simulink model "TRAMI_DCT_AT"  (R2018b)
settings: Solver=FixedStepDiscrete  StartTime=0.0  StopTime=88  FixedStep=10e-3  RelTol=1e-3  EnableMultiTasking=on
undefined symbols (not defined in the file): CONST_AP_GEAR_SUB_NEWTRAL, CONST_AP_IDLE_SPEED_CONT, CONST_AP_LOAD_SFT, CONST_AP_LOAD_SFT_HYS, CONST_CAR_WEIGHT, CONST_CL_NUM, CONST_F_DOWN_SYNCHRO, CONST_F_SYNCHRO, CONST_F_UP_SYNCHRO, CONST_FGR, CONST_I_FlYWHEEL, CONST_INATIA_CLANK, CONST_R_SHIFT_END_CD, CONST_R_SHIFT_END_EG, CONST_R_SHIFT_END_TD, CONST_R_SHIFT_END_UP, CONST_R_SYNCHRO_ENGAGE, CONST_R_TIRE, CONST_RATIO_TQ_REDUCTION, CONST_SKIP_SHIFT_MAX, CONST_SYN_NUM, CONST_T_SFT_END_EN, CONST_T_SFT_END_JUDGE, CONST_T_SFT_END_MAX, CONST_T_SFT_END_MIN, CONST_T_SHIFT_WAIT, CONST_T_TQ_PHASE_CD, CONST_T_TQ_PHASE_ND, CONST_T_TQ_PHASE_NR, CONST_T_TQ_PHASE_TD, CONST_T_TQ_PHASE_UP, CONST_TQ_CREEP_CONT, CONST_TQ_ENGAGE_CL_MARGIN, CONST_TQ_ENGAGE_CL_MIN, CONST_TQ_INATIA_TD_SHIFT, CONST_TQ_LOAD_SFT, CONST_TQ_LOAD_SFT_HYS, CONST_TQ_ND_ENGAGE, CONST_TQ_NR_ENGAGE, CONST_TQ_TQPHASE_MIN, CONST_V_IDLE_SPEED_CONT, Eng, FALSE, GrNP, GrRev, LoopTime, MAT_CL_ENGAGE, MAT_CL_SHARE_RATE, MAT_I_ACTUATOR, MAT_SYNCHRO_COM, MAT_T_GEAR_SUB_NEWTRAL, MAT_TRANS_MGR, MaxCL, Nm, PI, Shift_CD, Shift_ND, Shift_NR, Shift_TD, Shift_Up ... (+168)
libraries: simulink x26
(part 3 of 6)

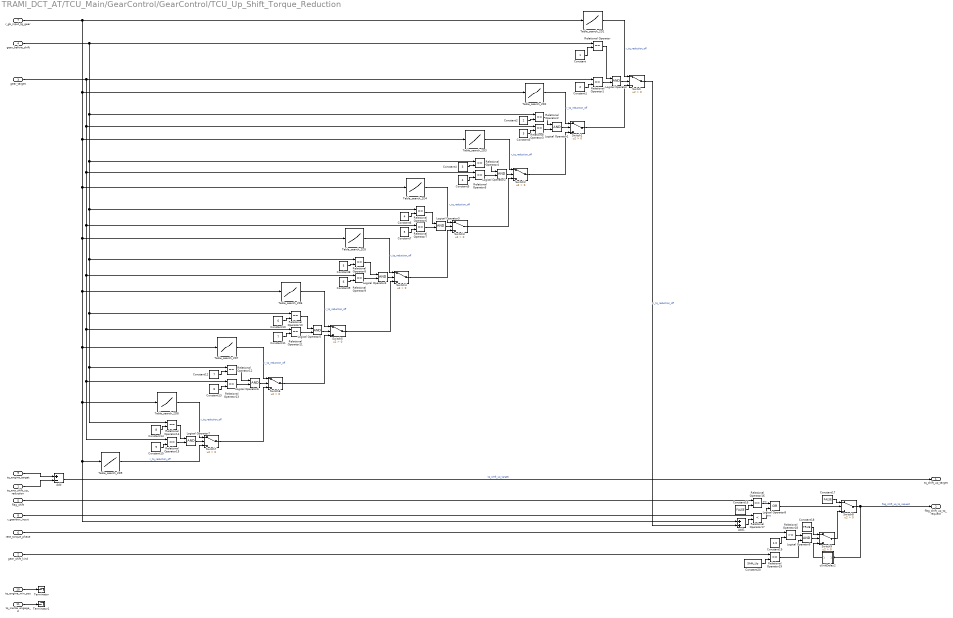
== system TRAMI_DCT_AT/TCU_Main/GearControl/GearControl/TCU_Up_Shift_Torque_Reduction ==
  tq_eng_shift_up_reduction : Inport  OutDataTypeStr=single
      settings: AttributesFormatString=アップシフト時のエンジントルクリダクション量[Nm]
  gear_shift_kind : Inport  Port=2  OutDataTypeStr=int16
      settings: AttributesFormatString=|
      | ギヤ変速種別
      | 5 : N->R
      | 4 : N->D
      | 3 : Torque demand shift
      | 2 : Coast down shift
      | 1 : Schedule up shift
      | [-]
  gear_target : Inport  Port=3  OutDataTypeStr=int16
      settings: AttributesFormatString=目標ギヤ段[-]
  gear_before_shift : Inport  Port=4  OutDataTypeStr=int16
      settings: AttributesFormatString=変速前ギヤ段[-]
  flag_shift : Inport  Port=5  OutDataTypeStr=boolean
      settings: AttributesFormatString=シフトフラグ[-]
  rate_torque_phase : Inport  Port=6  OutDataTypeStr=single
      settings: AttributesFormatString=トルクフェイズ移行比率[-]
  r_gb_input_tg_gear : Inport  Port=7  OutDataTypeStr=single
      settings: AttributesFormatString=|
      | 目標ギヤ段でのGearBox入力回転
      | （GearBox出力回転から演算)[rpm]
  r_gearbox_input : Inport  Port=8  OutDataTypeStr=single
      settings: AttributesFormatString=Gearbox input speed[rpm]
  tq_engine_target : Inport  Port=9  OutDataTypeStr=single
      settings: AttributesFormatString=目標エンジントルク[Nm]
  tq_engine_min_pos : Inport  ClipboardFcn=Eng.出力可能最小トルク[Nm]  Port=10  OutDataTypeStr=single
      settings: AttributesFormatString=Eng.出力可能最小トルク[Nm]
  tq_inertia_engage_cl : Inport  Port=11  OutDataTypeStr=single
      settings: AttributesFormatString=締結クラッチのイナーシャトルク[Nm]
  Add : Sum  Inputs=+-  OutDataTypeStr=single
  Add1 : Sum  OutDataTypeStr=single
  Constant : Constant  OutDataTypeStr=int16
  Constant1 : Constant  Value=2  OutDataTypeStr=int16
  Constant10 : Constant  Value=6  OutDataTypeStr=int16
  Constant11 : Constant  Value=7  OutDataTypeStr=int16
  Constant12 : Constant  Value=7  OutDataTypeStr=int16
  Constant13 : Constant  Value=8  OutDataTypeStr=int16
  Constant14 : Constant  Value=8  OutDataTypeStr=int16
  Constant15 : Constant  Value=9  OutDataTypeStr=int16
  Constant16 : Constant  Value=FALSE  OutDataTypeStr=boolean
  Constant17 : Constant  Value=FALSE  OutDataTypeStr=boolean
  Constant18 : Constant  Value=TRUE  OutDataTypeStr=boolean
  Constant19 : Constant  Value=1.0  OutDataTypeStr=single
  Constant2 : Constant  Value=2  OutDataTypeStr=int16
  Constant20 : Constant  Value=Shift_Up  OutDataTypeStr=single
  Constant3 : Constant  Value=3  OutDataTypeStr=int16
  Constant4 : Constant  Value=3  OutDataTypeStr=int16
  Constant5 : Constant  Value=4  OutDataTypeStr=int16
  Constant6 : Constant  Value=4  OutDataTypeStr=int16
  Constant7 : Constant  Value=5  OutDataTypeStr=int16
  Constant8 : Constant  Value=5  OutDataTypeStr=int16
  Constant9 : Constant  Value=6  OutDataTypeStr=int16
  Logical Operator{,1..7,9} (9 alike) : Logic  AllPortsSameDT=off  OutDataTypeStr=boolean
  Logical Operator8 : Logic  Operator=OR  AllPortsSameDT=off  OutDataTypeStr=boolean
  Relational Operator{,1..16,19} (18 alike) : RelationalOperator  Operator===  OutDataTypeStr=boolean  RndMeth=Nearest
  Relational Operator17 : RelationalOperator  Operator=<  OutDataTypeStr=boolean  RndMeth=Nearest
  Relational Operator18 : RelationalOperator  OutDataTypeStr=boolean  RndMeth=Nearest
  Switch{,1..7} (8 alike) : Switch  Criteria=u2 > Threshold  OutDataTypeStr=single
  Switch8 : Switch  Criteria=u2 > Threshold  OutDataTypeStr=boolean
  Switch9 : Switch  Criteria=u2 > Threshold  OutDataTypeStr=boolean
  Table_search_2D1 : Lookup_n-D  NumberOfTableDimensions=1  BreakpointsForDimension1=T2D_TQ_RED_OFF_12_X  Table=T2D_TQ_RED_OFF_12_Y  TableDataTypeStr=single  ExtrapMethod=Clip  UseLastTableValue=on  InternalRulePriority=Speed  OutDataTypeStr=single  RndMeth=Simplest  InputSameDT=on
      settings: AttributesFormatString=|
      | tbl = %<Table>
      | axis = %<BreakpointsForDimension1>
  Table_search_2D2 : Lookup_n-D  NumberOfTableDimensions=1  BreakpointsForDimension1=T2D_TQ_RED_OFF_23_X  Table=T2D_TQ_RED_OFF_23_Y  TableDataTypeStr=single  ExtrapMethod=Clip  UseLastTableValue=on  InternalRulePriority=Speed  OutDataTypeStr=single  RndMeth=Simplest  InputSameDT=on
      settings: AttributesFormatString=|
      | tbl = %<Table>
      | axis = %<BreakpointsForDimension1>
  Table_search_2D3 : Lookup_n-D  NumberOfTableDimensions=1  BreakpointsForDimension1=T2D_TQ_RED_OFF_34_X  Table=T2D_TQ_RED_OFF_34_Y  TableDataTypeStr=single  ExtrapMethod=Clip  UseLastTableValue=on  InternalRulePriority=Speed  OutDataTypeStr=single  RndMeth=Simplest  InputSameDT=on
      settings: AttributesFormatString=|
      | tbl = %<Table>
      | axis = %<BreakpointsForDimension1>
  Table_search_2D4 : Lookup_n-D  NumberOfTableDimensions=1  BreakpointsForDimension1=T2D_TQ_RED_OFF_45_X  Table=T2D_TQ_RED_OFF_45_Y  TableDataTypeStr=single  ExtrapMethod=Clip  UseLastTableValue=on  InternalRulePriority=Speed  OutDataTypeStr=single  RndMeth=Simplest  InputSameDT=on
      settings: AttributesFormatString=|
      | tbl = %<Table>
      | axis = %<BreakpointsForDimension1>
  Table_search_2D5 : Lookup_n-D  NumberOfTableDimensions=1  BreakpointsForDimension1=T2D_TQ_RED_OFF_56_X  Table=T2D_TQ_RED_OFF_56_Y  TableDataTypeStr=single  ExtrapMethod=Clip  UseLastTableValue=on  InternalRulePriority=Speed  OutDataTypeStr=single  RndMeth=Simplest  InputSameDT=on
      settings: AttributesFormatString=|
      | tbl = %<Table>
      | axis = %<BreakpointsForDimension1>
  Table_search_2D6 : Lookup_n-D  NumberOfTableDimensions=1  BreakpointsForDimension1=T2D_TQ_RED_OFF_67_X  Table=T2D_TQ_RED_OFF_67_Y  TableDataTypeStr=single  ExtrapMethod=Clip  UseLastTableValue=on  InternalRulePriority=Speed  OutDataTypeStr=single  RndMeth=Simplest  InputSameDT=on
      settings: AttributesFormatString=|
      | tbl = %<Table>
      | axis = %<BreakpointsForDimension1>
  Table_search_2D7 : Lookup_n-D  NumberOfTableDimensions=1  BreakpointsForDimension1=T2D_TQ_RED_OFF_78_X  Table=T2D_TQ_RED_OFF_78_Y  TableDataTypeStr=single  ExtrapMethod=Clip  UseLastTableValue=on  InternalRulePriority=Speed  OutDataTypeStr=single  RndMeth=Simplest  InputSameDT=on
      settings: AttributesFormatString=|
      | tbl = %<Table>
      | axis = %<BreakpointsForDimension1>
  Table_search_2D8 : Lookup_n-D  NumberOfTableDimensions=1  BreakpointsForDimension1=T2D_TQ_RED_OFF_89_X  Table=T2D_TQ_RED_OFF_89_Y  TableDataTypeStr=single  ExtrapMethod=Clip  UseLastTableValue=on  InternalRulePriority=Speed  OutDataTypeStr=single  RndMeth=Simplest  InputSameDT=on
      settings: AttributesFormatString=|
      | tbl = %<Table>
      | axis = %<BreakpointsForDimension1>
  Table_search_2D9 : Lookup_n-D  NumberOfTableDimensions=1  BreakpointsForDimension1=T2D_TQ_RED_OFF_9A_X  Table=T2D_TQ_RED_OFF_9A_Y  TableDataTypeStr=single  ExtrapMethod=Clip  UseLastTableValue=on  InternalRulePriority=Speed  OutDataTypeStr=single  RndMeth=Simplest  InputSameDT=on
      settings: AttributesFormatString=|
      | tbl = %<Table>
      | axis = %<BreakpointsForDimension1>
  Terminator : Terminator
  Terminator1 : Terminator
  cUnitDelay2 : Subsystem  mask(resetable_unit_delay){initParam=0}
      mask prompts: initParam "初期化値"
      mask Display:
      | dpoly(1,[1,0],'z')
      | text(2,10,'R')
  tq_shift_up_target : Outport  OutDataTypeStr=single
      settings: AttributesFormatString=アップシフト時のエンジントルク目標値[Nm]
  flag_shift_up_tq_request : Outport  Port=2  OutDataTypeStr=boolean
      settings: AttributesFormatString=アップシフト時のトルクリダクション実行フラグ[-]
  wires:
  r_gb_input_tg_gear/1 -> Add1/1, Table_search_2D9/1, Table_search_2D8/1, Table_search_2D7/1, Table_search_2D6/1, Table_search_2D5/1, Table_search_2D4/1, Table_search_2D3/1, Table_search_2D2/1, Table_search_2D1/1
  Constant/1 -> Relational Operator/2
  Relational Operator/1 -> Logical Operator/1
  Constant1/1 -> Relational Operator1/2
  Relational Operator1/1 -> Logical Operator/2
  Logical Operator/1 -> Switch/2
  Table_search_2D1/1 -> Switch/1  "r_tq_reduction_off"
  Switch1/1 -> Switch/3
  Relational Operator3/1 -> Logical Operator1/2
  Constant3/1 -> Relational Operator3/2
  Relational Operator2/1 -> Logical Operator1/1
  Constant2/1 -> Relational Operator2/2
  Logical Operator1/1 -> Switch1/2
  Table_search_2D2/1 -> Switch1/1  "r_tq_reduction_off"
  Switch2/1 -> Switch1/3
  Logical Operator2/1 -> Switch2/2
  Constant4/1 -> Relational Operator4/2
  Relational Operator4/1 -> Logical Operator2/1
  Constant5/1 -> Relational Operator5/2
  Relational Operator5/1 -> Logical Operator2/2
  Table_search_2D3/1 -> Switch2/1  "r_tq_reduction_off"
  Switch3/1 -> Switch2/3
  Switch4/1 -> Switch3/3
  Table_search_2D4/1 -> Switch3/1  "r_tq_reduction_off"
  Relational Operator7/1 -> Logical Operator3/2
  Constant7/1 -> Relational Operator7/2
  Relational Operator6/1 -> Logical Operator3/1
  Constant6/1 -> Relational Operator6/2
  Logical Operator3/1 -> Switch3/2
  Logical Operator4/1 -> Switch4/2
  Constant8/1 -> Relational Operator8/2
  Relational Operator8/1 -> Logical Operator4/1
  Constant9/1 -> Relational Operator9/2
  Relational Operator9/1 -> Logical Operator4/2
  Table_search_2D5/1 -> Switch4/1  "r_tq_reduction_off"
  Switch5/1 -> Switch4/3
  Switch6/1 -> Switch5/3
  Table_search_2D6/1 -> Switch5/1  "r_tq_reduction_off"
  Relational Operator11/1 -> Logical Operator5/2
  Constant11/1 -> Relational Operator11/2
  Relational Operator10/1 -> Logical Operator5/1
  Constant10/1 -> Relational Operator10/2
  Logical Operator5/1 -> Switch5/2
  gear_target/1 -> Relational Operator11/1, Relational Operator13/1, Relational Operator15/1, Relational Operator9/1, Relational Operator7/1, Relational Operator5/1, Relational Operator3/1, Relational Operator1/1
  gear_before_shift/1 -> Relational Operator14/1, Relational Operator12/1, Relational Operator10/1, Relational Operator8/1, Relational Operator6/1, Relational Operator4/1, Relational Operator2/1, Relational Operator/1
  Logical Operator6/1 -> Switch6/2
  Constant12/1 -> Relational Operator12/2
  Relational Operator12/1 -> Logical Operator6/1
  Constant13/1 -> Relational Operator13/2
  Relational Operator13/1 -> Logical Operator6/2
  Table_search_2D7/1 -> Switch6/1  "r_tq_reduction_off"
  Switch7/1 -> Switch6/3
  Table_search_2D9/1 -> Switch7/3  "r_tq_reduction_off"
  Table_search_2D8/1 -> Switch7/1  "r_tq_reduction_off"
  Relational Operator15/1 -> Logical Operator7/2
  Constant15/1 -> Relational Operator15/2
  Relational Operator14/1 -> Logical Operator7/1
  Constant14/1 -> Relational Operator14/2
  Logical Operator7/1 -> Switch7/2
  tq_engine_target/1 -> Add/1
  tq_eng_shift_up_reduction/1 -> Add/2
  Add/1 -> tq_shift_up_target/1  "tq_shift_up_target"
  Constant16/1 -> Relational Operator16/2
  flag_shift/1 -> Relational Operator16/1
  Relational Operator16/1 -> Logical Operator8/1  "ans"
  Logical Operator8/1 -> Switch8/2
  Add1/1 -> Relational Operator17/2
  r_gearbox_input/1 -> Relational Operator17/1
  Switch/1 -> Add1/2  "r_tq_reduction_off"
  Relational Operator17/1 -> Logical Operator8/2  "ans"
  Constant17/1 -> Switch8/1
  rate_torque_phase/1 -> Relational Operator18/1
  Constant19/1 -> Relational Operator18/2
  Relational Operator18/1 -> Logical Operator9/1
  Logical Operator9/1 -> Switch9/2
  Switch9/1 -> Switch8/3
  Constant18/1 -> Switch9/1
  Switch8/1 -> flag_shift_up_tq_request/1, cUnitDelay2/1(<param>)  "flag_shift_up_tq_request"
  Relational Operator19/1 -> Logical Operator9/2
  cUnitDelay2/1(preParam) -> Switch9/3
  gear_shift_kind/1 -> Relational Operator19/1
  Constant20/1 -> Relational Operator19/2
  tq_engine_min_pos/1 -> Terminator/1
  tq_inertia_engage_cl/1 -> Terminator1/1

== system TRAMI_DCT_AT/TCU_Main/ShiftScheduleControl/ShiftScheduleControl/TCU_Gear_Shift_Type ==
  flag_load_shift : Inport  OutDataTypeStr=boolean
      settings: AttributesFormatString=Poweron判定[-]
  flag_shift : Inport  Port=2  OutDataTypeStr=boolean
      settings: AttributesFormatString=シフトフラグ[-]
  gear_target : Inport  Port=3  OutDataTypeStr=int16
      settings: AttributesFormatString=目標ギヤ段[-]
  gear_before_shift : Inport  Port=4  OutDataTypeStr=int16
      settings: AttributesFormatString=変速前ギヤ段[-]
  Constant : Constant  Value=0  OutDataTypeStr=int16
  Constant1 : Constant  Value=GrRev  OutDataTypeStr=int16
  Constant2 : Constant  Value=Shift_NR  OutDataTypeStr=int16
  Constant3 : Constant  Value=0  OutDataTypeStr=int16
  Constant4 : Constant  Value=Shift_ND  OutDataTypeStr=int16
  Constant5 : Constant  Value=Shift_Up  OutDataTypeStr=int16
  Constant6 : Constant  Value=Shift_TD  OutDataTypeStr=int16
  Constant7 : Constant  Value=Shift_CD  OutDataTypeStr=int16
  Logical Operator : Logic  AllPortsSameDT=off  OutDataTypeStr=boolean
  Relational Operator : RelationalOperator  Operator===  OutDataTypeStr=boolean  RndMeth=Nearest
  Relational Operator1 : RelationalOperator  Operator=>  OutDataTypeStr=boolean  RndMeth=Nearest
  Relational Operator2 : RelationalOperator  Operator=<=  OutDataTypeStr=boolean  RndMeth=Nearest
  Relational Operator3 : RelationalOperator  Operator=>  OutDataTypeStr=boolean  RndMeth=Nearest
  Relational Operator4 : RelationalOperator  Operator=<  OutDataTypeStr=boolean  RndMeth=Nearest
  Switch{,1..5} (6 alike) : Switch  Criteria=u2 > Threshold  OutDataTypeStr=int16
  cUnitDelay2 : Subsystem  mask(resetable_unit_delay){initParam=0}
      mask prompts: initParam "初期化値"
      mask Display:
      | dpoly(1,[1,0],'z')
      | text(2,10,'R')
  gear_shift_kind : Outport  OutDataTypeStr=int16
      settings: AttributesFormatString=|
      | ギヤ変速種別
      | 5 : N->R
      | 4 : N->D
      | 3 : Torque demand shift
      | 2 : Coast down shift
      | 1 : Schedule up shift
      | [-]
  wires:
  flag_load_shift/1 -> Switch5/2
  Constant/1 -> Switch/3
  Switch1/1 -> Switch/1
  Constant1/1 -> Relational Operator/2
  Relational Operator/1 -> Switch1/2
  Constant2/1 -> Switch1/1
  Switch2/1 -> Switch1/3
  Relational Operator1/1 -> Logical Operator/1
  Constant3/1 -> Relational Operator2/2, Relational Operator1/2
  gear_target/1 -> Relational Operator/1, Relational Operator1/1, Relational Operator4/1, Relational Operator3/1  "gear_target"
  Logical Operator/1 -> Switch2/2
  gear_before_shift/1 -> Relational Operator3/2, Relational Operator4/2, Relational Operator2/1  "gear_before_shift"
  Relational Operator2/1 -> Logical Operator/2
  Constant4/1 -> Switch2/1
  Relational Operator3/1 -> Switch3/2
  Constant5/1 -> Switch3/1
  Switch4/1 -> Switch3/3
  Switch3/1 -> Switch2/3
  Relational Operator4/1 -> Switch4/2
  cUnitDelay2/1(preParam) -> Switch4/3  "gear_shift_kind"
  Switch5/1 -> Switch4/1
  flag_shift/1 -> Switch/2  "flag_shift"
  Constant6/1 -> Switch5/1
  Constant7/1 -> Switch5/3
  Switch/1 -> cUnitDelay2/1(<param>), gear_shift_kind/1  "gear_shift_kind"

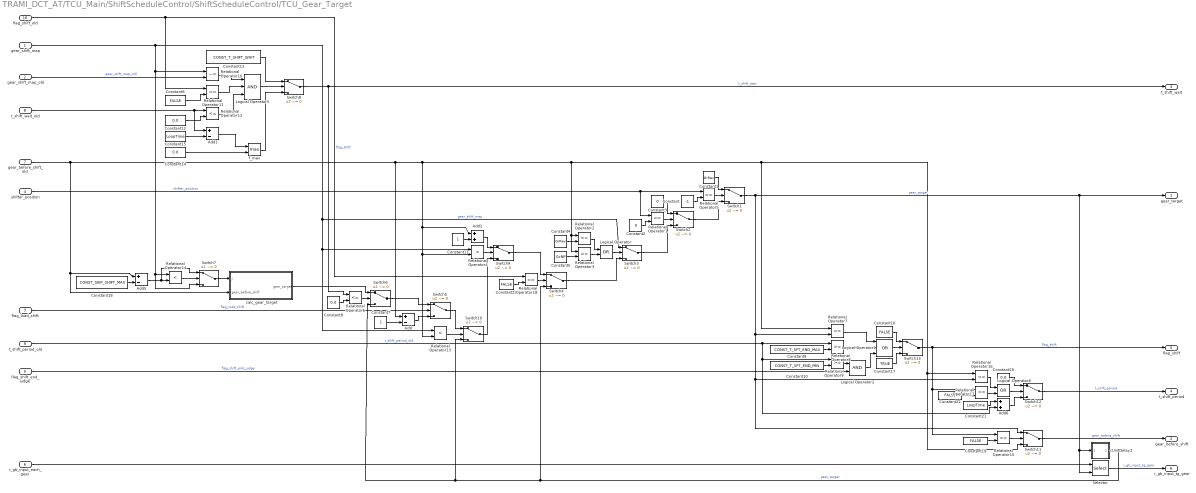
== system TRAMI_DCT_AT/TCU_Main/ShiftScheduleControl/ShiftScheduleControl/TCU_Gear_Target ==
  gear_shift_map : Inport  OutDataTypeStr=int16
      settings: AttributesFormatString=シフトマップから算出されるギヤ段[-]
  gear_shift_map_old : Inport  Port=2  OutDataTypeStr=int16
      settings: AttributesFormatString=前回のシフトマップから算出されるギヤ段[-]
  flag_load_shift : Inport  Port=3  OutDataTypeStr=boolean
      settings: AttributesFormatString=Poweron判定[-]
  shifter_position : Inport  Port=4  OutDataTypeStr=int16
      settings: AttributesFormatString=シフター位置[-]
  flag_shift_end_judge : Inport  Port=5  OutDataTypeStr=boolean
      settings: AttributesFormatString=変速終了フラグ[-]
  r_gb_input_each_gear : Inport  Port=6  OutDataTypeStr=single
      settings: AttributesFormatString=|
      | 各ギヤ段でのGearBox入力回転
      | 配列数12: 左から
      | N, 1st, 2nd, 3rd ,4th ,5th ,6th ,7th, 8th, 9th, 10th, Rev
      | [rpm]
  "  gear_before_shift_old" : Inport  Port=7  OutDataTypeStr=int16
      settings: AttributesFormatString=前回の変速前ギヤ段[-]
  "  t_shift_wait_old" : Inport  Port=8  OutDataTypeStr=single
      settings: AttributesFormatString=前回の変速判定待機時間[ms]
  "  t_shift_period_old" : Inport  Port=9  OutDataTypeStr=single
      settings: AttributesFormatString=前回変速制御時間[ms]
  "  flag_shift_old" : Inport  Port=10  OutDataTypeStr=boolean
      settings: AttributesFormatString=前回のシフトフラグ[-]
  Add : Sum  Inputs=+-  OutDataTypeStr=int16
  Add1 : Sum  Inputs=+-  OutDataTypeStr=single
  Add2 : Sum  OutDataTypeStr=int16
  Add5 : Sum  Inputs=+-  OutDataTypeStr=int16
  Add6 : Sum  OutDataTypeStr=single
  Constant : Constant  Value=-1  OutDataTypeStr=int16
  Constant1 : Constant  Value=GrRev  OutDataTypeStr=int16
  Constant10 : Constant  Value=CONST_T_SFT_END_MIN  OutDataTypeStr=int16
  Constant11 : Constant  OutDataTypeStr=int16
  Constant{8,12,14,20} (4 alike) : Constant  Value=0.0  OutDataTypeStr=single
  Constant13 : Constant  Value=CONST_T_SHIFT_WAIT  OutDataTypeStr=single
  Constant15 : Constant  Value=LoopTime  OutDataTypeStr=single
  Constant16 : Constant  Value=FALSE  OutDataTypeStr=boolean
  Constant17 : Constant  Value=TRUE  OutDataTypeStr=boolean
  Constant18 : Constant  Value=CONST_SKIP_SHIFT_MAX  OutDataTypeStr=int16
  Constant19 : Constant  Value=FALSE  OutDataTypeStr=int16
  Constant2 : Constant  Value=0  OutDataTypeStr=int16
  Constant21 : Constant  Value=LoopTime  OutDataTypeStr=single
  Constant22 : Constant  Value=FALSE  OutDataTypeStr=int16
  Constant23 : Constant  Value=FALSE  OutDataTypeStr=boolean
  Constant3 : Constant  Value=0  OutDataTypeStr=int16
  Constant4 : Constant  Value=GrRev  OutDataTypeStr=int16
  Constant5 : Constant  Value=GrNP  OutDataTypeStr=int16
  Constant6 : Constant  Value=FALSE  OutDataTypeStr=boolean
  Constant7 : Constant  OutDataTypeStr=int16
  Constant9 : Constant  Value=CONST_T_SFT_END_MAX  OutDataTypeStr=int16
  Logical Operator : Logic  Operator=OR  AllPortsSameDT=off  OutDataTypeStr=boolean
  Logical Operator1 : Logic  Operator=OR  Inputs=3  AllPortsSameDT=off  OutDataTypeStr=boolean
  Logical Operator2 : Logic  AllPortsSameDT=off  OutDataTypeStr=boolean
  Logical Operator5 : Logic  Inputs=3  AllPortsSameDT=off  OutDataTypeStr=boolean
  Logical Operator6 : Logic  Operator=OR  AllPortsSameDT=off  OutDataTypeStr=boolean
  Relational Operator{1..3,5,7,11,15..18} (10 alike) : RelationalOperator  Operator===  OutDataTypeStr=boolean  RndMeth=Nearest
  Relational Operator10 : RelationalOperator  Operator=~=  OutDataTypeStr=boolean  RndMeth=Nearest
  Relational Operator12 : RelationalOperator  Operator=<=  OutDataTypeStr=boolean  RndMeth=Nearest
  Relational Operator13 : RelationalOperator  Operator=<  OutDataTypeStr=boolean  RndMeth=Nearest
  Relational Operator14 : RelationalOperator  Operator=<  OutDataTypeStr=boolean  RndMeth=Nearest
  Relational Operator4 : RelationalOperator  Operator=>  OutDataTypeStr=boolean  RndMeth=Nearest
  Relational Operator6 : RelationalOperator  Operator=<=  OutDataTypeStr=boolean  RndMeth=Nearest
  Relational Operator8 : RelationalOperator  OutDataTypeStr=boolean  RndMeth=Nearest
  Relational Operator9 : RelationalOperator  OutDataTypeStr=boolean  RndMeth=Nearest
  Selector : Selector  IndexMode=Zero-based  InputPortWidth=12  IndexOptions=Index vector (port)  Indices=[1 3]  OutputSizes=1
  Switch{1..7,9..11} (10 alike) : Switch  Criteria=u2 ~= 0  OutDataTypeStr=int16
  Switch12 : Switch  Criteria=u2 ~= 0  OutDataTypeStr=single
  Switch13 : Switch  Criteria=u2 ~= 0  OutDataTypeStr=boolean
  Switch8 : Switch  Criteria=u2 ~= 0  OutDataTypeStr=single
  cUnitDelay2 : Subsystem  mask(resetable_unit_delay){initParam=0}
      mask prompts: initParam "初期化値"
      mask Display:
      | dpoly(1,[1,0],'z')
      | text(2,10,'R')
  calc_gear_target : Subsystem
  f_max : MinMax  Function=max  Inputs=2  OutDataTypeStr=single
  gear_target : Outport  OutDataTypeStr=int16
      settings: AttributesFormatString=目標ギヤ段[-]
  gear_before_shift : Outport  Port=2  OutDataTypeStr=int16
      settings: AttributesFormatString=変速前ギヤ段[-]
  t_shift_wait : Outport  Port=3  OutDataTypeStr=single
      settings: AttributesFormatString=変速判定待機時間[ms]
  t_shift_period : Outport  Port=4  OutDataTypeStr=single
      settings: AttributesFormatString=変速制御時間[ms]
  flag_shift : Outport  Port=5  OutDataTypeStr=boolean
      settings: AttributesFormatString=シフトフラグ[-]
  r_gb_input_tg_gear : Outport  Port=6  OutDataTypeStr=single
      settings: AttributesFormatString=目標ギヤ段によるGearBox入力回転[rpm]
  wires:
  Switch12/1 -> t_shift_period/1  "t_shift_period"
  Switch11/1 -> gear_before_shift/1  "gear_before_shift"
  cUnitDelay2/1(preParam) -> Switch6/3, Switch10/3, Switch4/3  "gear_target"
  Selector/1 -> r_gb_input_tg_gear/1  "r_gb_input_tg_gear"
  Add1/1 -> f_max/1
  "  gear_before_shift_old"/1 -> Relational Operator13/2, Relational Operator4/2, Add2/1, Relational Operator3/1, Relational Operator2/1, Relational Operator16/1, Switch11/3, Relational Operator7/1, Add/1, calc_gear_target/2(gear_before_shift), Add5/1
  Switch13/1 -> flag_shift/1, Relational Operator17/1, Relational Operator15/1  "flag_shift"
  Constant17/1 -> Switch13/3
  Constant16/1 -> Switch13/1
  Switch8/1 -> t_shift_wait/1, Relational Operator6/1  "t_shift_wait"
  Switch10/1 -> Switch9/3
  Constant23/1 -> Relational Operator18/2
  Constant22/1 -> Relational Operator17/2
  Relational Operator16/1 -> Logical Operator6/1
  Relational Operator17/1 -> Logical Operator6/2
  Logical Operator6/1 -> Switch12/2
  Add6/1 -> Switch12/3
  Constant21/1 -> Add6/1
  "  t_shift_period_old"/1 -> Relational Operator8/1, Relational Operator9/1, Add6/2  "t_shift_period_old"
  Constant20/1 -> Switch12/1
  Constant19/1 -> Relational Operator15/2
  Relational Operator15/1 -> Switch11/2
  r_gb_input_each_gear/1 -> Selector/1
  Add5/1 -> Switch7/1, Relational Operator14/2
  Constant18/1 -> Add5/2
  Relational Operator14/1 -> Switch7/2
  Switch5/1 -> Switch10/1
  Relational Operator13/1 -> Switch10/2
  Constant11/1 -> Add2/2
  Add2/1 -> Switch9/1
  Relational Operator4/1 -> Switch9/2
  Switch9/1 -> Switch4/1
  Constant15/1 -> Add1/2
  Constant14/1 -> f_max/2
  Constant12/1 -> Relational Operator12/2
  f_max/1 -> Switch8/3
  Constant13/1 -> Switch8/1
  Logical Operator5/1 -> Switch8/2
  Relational Operator12/1 -> Logical Operator5/3
  Relational Operator11/1 -> Logical Operator5/2
  Constant6/1 -> Relational Operator11/2
  Relational Operator10/1 -> Logical Operator5/1
  gear_shift_map_old/1 -> Relational Operator10/2  "gear_shift_map_old"
  "  flag_shift_old"/1 -> Relational Operator11/1, Relational Operator18/1  "flag_shift"
  Relational Operator18/1 -> Switch4/2
  Switch7/1 -> calc_gear_target/1(j)
  Logical Operator1/1 -> Switch13/2
  Logical Operator2/1 -> Logical Operator1/3
  flag_shift_end_judge/1 -> Logical Operator2/2  "flag_shift_end_judge"
  Constant10/1 -> Relational Operator9/2
  Relational Operator9/1 -> Logical Operator2/1
  Constant9/1 -> Relational Operator8/2
  Relational Operator8/1 -> Logical Operator1/2
  Switch1/1 -> gear_target/1, cUnitDelay2/1(<param>), Selector/2, Switch11/1, Relational Operator16/2, Relational Operator7/2  "gear_target"
  Relational Operator7/1 -> Logical Operator1/1
  gear_shift_map/1 -> Relational Operator14/1, Switch7/3, Relational Operator10/1, Relational Operator13/1, Relational Operator4/1, Switch3/1  "gear_shift_map"
  calc_gear_target/1(gear_target) -> Switch6/1
  Constant8/1 -> Relational Operator6/2
  "  t_shift_wait_old"/1 -> Relational Operator12/1, Add1/1
  Relational Operator6/1 -> Switch6/2
  Switch6/1 -> Switch5/1
  Constant7/1 -> Add/2
  Add/1 -> Switch5/3
  flag_load_shift/1 -> Switch5/2  "flag_load_shift"
  Switch4/1 -> Switch3/3
  Constant5/1 -> Relational Operator3/2
  Relational Operator3/1 -> Logical Operator/2
  Constant4/1 -> Relational Operator2/2
  Relational Operator2/1 -> Logical Operator/1
  Logical Operator/1 -> Switch3/2
  Switch3/1 -> Switch2/3
  Constant3/1 -> Switch2/1
  Constant2/1 -> Relational Operator1/2
  Relational Operator1/1 -> Switch2/2
  Switch2/1 -> Switch1/3
  Constant1/1 -> Switch1/1
  Relational Operator5/1 -> Switch1/2
  Constant/1 -> Relational Operator5/2
  shifter_position/1 -> Relational Operator1/1, Relational Operator5/1  "shifter_position"

== system TRAMI_DCT_AT/TCU_Main/ShiftScheduleControl/ShiftScheduleControl/TCU_Load_shift ==
  flag_load_shift_old : Inport  OutDataTypeStr=boolean
      settings: AttributesFormatString=前回Poweron判定[-]
  flag_ap_load_shift_old : Inport  Port=2  OutDataTypeStr=boolean
      settings: AttributesFormatString=前回Poweron判定アクセル開度[-]
  flag_tq_load_shift_old : Inport  Port=3  OutDataTypeStr=boolean
      settings: AttributesFormatString=前回Poweron判定エンジントルク[-]
  accel_position : Inport  Port=4  OutDataTypeStr=single
      settings: AttributesFormatString=アクセル開度[%]
  tq_engine_target : Inport  Port=5  OutDataTypeStr=single
      settings: AttributesFormatString=目標エンジントルク[Nm]
  Constant : Constant  Value=CONST_AP_LOAD_SFT  OutDataTypeStr=single
  Constant1 : Constant  Value=CONST_AP_LOAD_SFT_HYS  OutDataTypeStr=single
  Constant2 : Constant  Value=CONST_TQ_LOAD_SFT  OutDataTypeStr=single
  Constant3 : Constant  Value=CONST_TQ_LOAD_SFT_HYS  OutDataTypeStr=single
  Constant5 : Constant  Value=FALSE  OutDataTypeStr=boolean
  Constant6 : Constant  Value=TRUE  OutDataTypeStr=boolean
  Logical Operator4 : Logic  Operator=OR  AllPortsSameDT=off  OutDataTypeStr=boolean
  Switch2 : Switch  Criteria=u2 ~= 0  OutDataTypeStr=boolean
  Switch_with_hys : Subsystem
      settings: AttributesFormatString=ヒス付きソフトスイッチ関数
  Switch_with_hys1 : Subsystem
      settings: AttributesFormatString=ヒス付きソフトスイッチ関数
  Terminator : Terminator
  flag_load_shift : Outport  OutDataTypeStr=boolean
      settings: AttributesFormatString=Poweron判定[-]
  flag_ap_load_shift : Outport  Port=2  OutDataTypeStr=boolean
      settings: AttributesFormatString=Poweron判定アクセル開度[-]
  flag_tq_load_shift : Outport  Port=3  OutDataTypeStr=boolean
      settings: AttributesFormatString=Poweron判定エンジントルク[-]
  wires:
  accel_position/1 -> Switch_with_hys/2(val)
  Constant/1 -> Switch_with_hys/3(cal)
  Constant2/1 -> Switch_with_hys1/3(cal)
  Constant1/1 -> Switch_with_hys/4(hys)
  Constant3/1 -> Switch_with_hys1/4(hys)
  Switch_with_hys/1(flag) -> Logical Operator4/1, flag_ap_load_shift/1  "flag_ap_load_shift"
  Logical Operator4/1 -> Switch2/2
  Constant6/1 -> Switch2/1
  Constant5/1 -> Switch2/3
  Switch_with_hys1/1(flag) -> flag_tq_load_shift/1, Logical Operator4/2  "flag_tq_load_shift"
  Switch2/1 -> flag_load_shift/1  "flag_load_shift"
  tq_engine_target/1 -> Switch_with_hys1/2(val)
  flag_ap_load_shift_old/1 -> Switch_with_hys/1(flag_old)
  flag_tq_load_shift_old/1 -> Switch_with_hys1/1(flag_old)
  flag_load_shift_old/1 -> Terminator/1

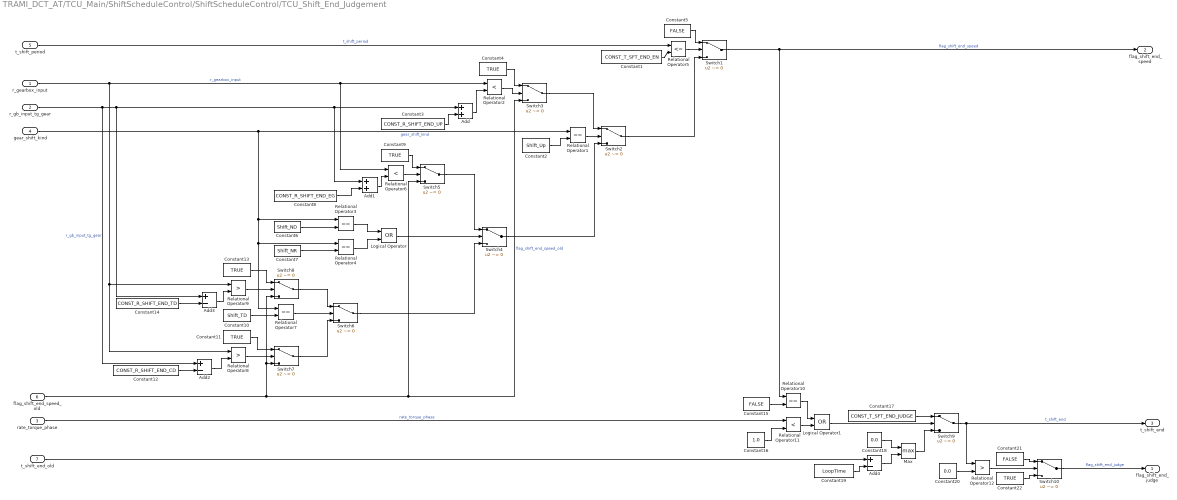
== system TRAMI_DCT_AT/TCU_Main/ShiftScheduleControl/ShiftScheduleControl/TCU_Shift_End_Judgement ==
  r_gearbox_input : Inport  OutDataTypeStr=single
      settings: AttributesFormatString=Geabox input speed[rpm]
  r_gb_input_tg_gear : Inport  Port=2  OutDataTypeStr=single
      settings: AttributesFormatString=目標ギヤ段によるGearBox入力回転[rpm]
  rate_torque_phase : Inport  Port=3  OutDataTypeStr=single
      settings: AttributesFormatString=トルクフェイズ移行比率[-]
  gear_shift_kind : Inport  Port=4  OutDataTypeStr=int16
      settings: AttributesFormatString=|
      | ギヤ変速種別
      | 5 : N->R
      | 4 : N->D
      | 3 : Torque demand shift
      | 2 : Coast down shift
      | 1 : Schedule up shift
      | [-]
  t_shift_period : Inport  Port=5  OutDataTypeStr=single
      settings: AttributesFormatString=変速制御時間[ms]
  flag_shift_end_speed_old : Inport  Port=6  OutDataTypeStr=boolean
      settings: AttributesFormatString=前回の回転による変速終了判定フラグ[-]
  t_shift_end_old : Inport  Port=7  OutDataTypeStr=single
      settings: AttributesFormatString=前回の変速終了判定タイマー[ms]
  Add : Sum  OutDataTypeStr=single
  Add1 : Sum  AccumDataTypeStr=int16  OutDataTypeStr=single
  Add2 : Sum  Inputs=+-  OutDataTypeStr=single
  Add3 : Sum  Inputs=+-  AccumDataTypeStr=single  OutDataTypeStr=single
  Add4 : Sum  Inputs=+-  OutDataTypeStr=single
  Constant1 : Constant  Value=CONST_T_SFT_END_EN  OutDataTypeStr=single
  Constant10 : Constant  Value=Shift_TD  OutDataTypeStr=int16
  Constant{4,9,11,13,22} (5 alike) : Constant  Value=TRUE  OutDataTypeStr=boolean
  Constant12 : Constant  Value=CONST_R_SHIFT_END_CD  OutDataTypeStr=single
  Constant14 : Constant  Value=CONST_R_SHIFT_END_TD  OutDataTypeStr=single
  Constant15 : Constant  Value=FALSE  OutDataTypeStr=boolean
  Constant16 : Constant  Value=1.0  OutDataTypeStr=single
  Constant17 : Constant  Value=CONST_T_SFT_END_JUDGE  OutDataTypeStr=single
  Constant18 : Constant  Value=0.0  OutDataTypeStr=single
  Constant19 : Constant  Value=LoopTime  OutDataTypeStr=single
  Constant2 : Constant  Value=Shift_Up  OutDataTypeStr=int16
  Constant20 : Constant  Value=0.0  OutDataTypeStr=single
  Constant21 : Constant  Value=FALSE  OutDataTypeStr=boolean
  Constant3 : Constant  Value=CONST_R_SHIFT_END_UP  OutDataTypeStr=single
  Constant5 : Constant  Value=FALSE  OutDataTypeStr=boolean
  Constant6 : Constant  Value=Shift_ND  OutDataTypeStr=int16
  Constant7 : Constant  Value=Shift_NR  OutDataTypeStr=int16
  Constant8 : Constant  Value=CONST_R_SHIFT_END_EG  VectorParams1D=off  OutDataTypeStr=single
  Logical Operator : Logic  Operator=OR  AllPortsSameDT=off  OutDataTypeStr=boolean
  Logical Operator1 : Logic  Operator=OR  AllPortsSameDT=off  OutDataTypeStr=boolean
  Max : MinMax  Function=max  Inputs=2  OutDataTypeStr=single
  Relational Operator{1,3..4,7,10} (5 alike) : RelationalOperator  Operator===  OutDataTypeStr=boolean  RndMeth=Nearest
  Relational Operator11 : RelationalOperator  Operator=<  OutDataTypeStr=boolean  RndMeth=Nearest
  Relational Operator12 : RelationalOperator  Operator=>  OutDataTypeStr=boolean  RndMeth=Nearest
  Relational Operator2 : RelationalOperator  Operator=<  OutDataTypeStr=boolean  RndMeth=Nearest
  Relational Operator5 : RelationalOperator  Operator=<=  OutDataTypeStr=boolean  RndMeth=Nearest
  Relational Operator6 : RelationalOperator  Operator=<  OutDataTypeStr=boolean  RndMeth=Nearest
  Relational Operator8 : RelationalOperator  Operator=>  OutDataTypeStr=boolean  RndMeth=Nearest
  Relational Operator9 : RelationalOperator  Operator=>  OutDataTypeStr=boolean  RndMeth=Nearest
  Switch{1..8,10} (9 alike) : Switch  Criteria=u2 ~= 0  OutDataTypeStr=boolean
  Switch9 : Switch  Criteria=u2 ~= 0  OutDataTypeStr=single
  flag_shift_end_judge : Outport  OutDataTypeStr=boolean
      settings: AttributesFormatString=変速終了フラグ[-]
  flag_shift_end_speed : Outport  Port=2  OutDataTypeStr=boolean
      settings: AttributesFormatString=回転による変速終了判定フラグ[-]
  t_shift_end : Outport  Port=3  OutDataTypeStr=single
      settings: AttributesFormatString=変速終了判定タイマー[ms]
  wires:
  Relational Operator5/1 -> Switch1/2
  Constant1/1 -> Relational Operator5/2
  Switch1/1 -> flag_shift_end_speed/1, Relational Operator10/1  "flag_shift_end_speed"
  Constant5/1 -> Switch1/1
  t_shift_period/1 -> Relational Operator5/1  "t_shift_period"
  Switch2/1 -> Switch1/3
  Constant2/1 -> Relational Operator1/2
  Relational Operator1/1 -> Switch2/2
  gear_shift_kind/1 -> Relational Operator7/1, Relational Operator4/1, Relational Operator3/1, Relational Operator1/1  "gear_shift_kind"
  Switch3/1 -> Switch2/1
  Switch4/1 -> Switch2/3
  Relational Operator2/1 -> Switch3/2
  Constant4/1 -> Switch3/1
  Add/1 -> Relational Operator2/2
  r_gearbox_input/1 -> Relational Operator8/1, Relational Operator9/1, Relational Operator6/1, Relational Operator2/1  "r_gearbox_input"
  r_gb_input_tg_gear/1 -> Add/1, Add1/1, Add3/1, Add2/1  "r_gb_input_tg_gear"
  Constant3/1 -> Add/2
  Logical Operator/1 -> Switch4/2
  Relational Operator3/1 -> Logical Operator/1
  Constant6/1 -> Relational Operator3/2
  Relational Operator4/1 -> Logical Operator/2
  Constant7/1 -> Relational Operator4/2
  Switch5/1 -> Switch4/1
  Constant8/1 -> Add1/2
  Relational Operator6/1 -> Switch5/2
  Add1/1 -> Relational Operator6/2
  Constant9/1 -> Switch5/1
  Switch6/1 -> Switch4/3
  Relational Operator7/1 -> Switch6/2
  Constant10/1 -> Relational Operator7/2
  Switch7/1 -> Switch6/3
  flag_shift_end_speed_old/1 -> Switch3/3, Switch5/3, Switch7/3, Switch8/3  "flag_shift_end_speed_old"
  Constant11/1 -> Switch7/1
  Add2/1 -> Relational Operator8/2
  Constant12/1 -> Add2/2
  Switch8/1 -> Switch6/1
  Constant13/1 -> Switch8/1
  Add3/1 -> Relational Operator9/2
  Constant14/1 -> Add3/2
  Relational Operator8/1 -> Switch7/2
  Relational Operator9/1 -> Switch8/2
  Constant15/1 -> Relational Operator10/2
  Relational Operator10/1 -> Logical Operator1/1
  rate_torque_phase/1 -> Relational Operator11/1  "rate_torque_phase"
  Constant16/1 -> Relational Operator11/2
  Relational Operator11/1 -> Logical Operator1/2
  Logical Operator1/1 -> Switch9/2
  Constant17/1 -> Switch9/1
  Switch9/1 -> t_shift_end/1, Relational Operator12/1  "t_shift_end"
  Max/1 -> Switch9/3
  Constant18/1 -> Max/1
  t_shift_end_old/1 -> Add4/1
  Add4/1 -> Max/2
  Constant19/1 -> Add4/2
  Constant20/1 -> Relational Operator12/2
  Relational Operator12/1 -> Switch10/2
  Constant21/1 -> Switch10/1
  Constant22/1 -> Switch10/3
  Switch10/1 -> flag_shift_end_judge/1  "flag_shift_end_judge"

== system TRAMI_DCT_AT/TCU_Main/ShiftScheduleControl/ShiftScheduleControl/TCU_Shift_Schedule ==
  gear_shift_map_old : Inport  OutDataTypeStr=int16
      settings: AttributesFormatString=前回のシフトマップから算出されるギヤ段の値[-]
  shifter_position : Inport  Port=2  OutDataTypeStr=int16
      settings: AttributesFormatString=|
      | シフター位置[-]
      | (Rev=-1; N=0 ; D=1)
  accel_position : Inport  Port=3  OutDataTypeStr=single
      settings: AttributesFormatString=アクセル開度[%]
  v_vehicle : Inport  Port=4  OutDataTypeStr=single
      settings: AttributesFormatString=車速[km/h]
  Constant : Constant  Value=-1  OutDataTypeStr=int16
  Constant1 : Constant  Value=GrRev  OutDataTypeStr=int16
  Constant2 : Constant  OutDataTypeStr=int16
  Relational Operator : RelationalOperator  Operator===  OutDataTypeStr=boolean  RndMeth=Nearest
  Subsystem : Subsystem
  Subsystem1 : Subsystem
  Subsystem2 : Subsystem
  Subsystem3 : Subsystem
  Subsystem4 : Subsystem
  Subsystem5 : Subsystem
  Subsystem6 : Subsystem
  Subsystem7 : Subsystem
  Subsystem8 : Subsystem
  Switch2 : Switch  Criteria=u2 ~= 0  OutDataTypeStr=int16
  Table_search_2D1 : Lookup_n-D  NumberOfTableDimensions=1  BreakpointsForDimension1=T2D_V_SFT_A9_X  Table=T2D_V_SFT_A9_Y  TableDataTypeStr=single  ExtrapMethod=Clip  UseLastTableValue=on  InternalRulePriority=Speed  OutDataTypeStr=single  RndMeth=Simplest  InputSameDT=on
      settings: AttributesFormatString=|
      | tbl = %<Table>
      | axis = %<BreakpointsForDimension1>
  Table_search_2D10 : Lookup_n-D  NumberOfTableDimensions=1  BreakpointsForDimension1=T2D_V_SFT_9A_X  Table=T2D_V_SFT_9A_Y  TableDataTypeStr=single  ExtrapMethod=Clip  UseLastTableValue=on  InternalRulePriority=Speed  OutDataTypeStr=single  RndMeth=Simplest  InputSameDT=on
      settings: AttributesFormatString=|
      | tbl = %<Table>
      | axis = %<BreakpointsForDimension1>
  Table_search_2D11 : Lookup_n-D  NumberOfTableDimensions=1  BreakpointsForDimension1=T2D_V_SFT_89_X  Table=T2D_V_SFT_89_Y  TableDataTypeStr=single  ExtrapMethod=Clip  UseLastTableValue=on  InternalRulePriority=Speed  OutDataTypeStr=single  RndMeth=Simplest  InputSameDT=on
      settings: AttributesFormatString=|
      | tbl = %<Table>
      | axis = %<BreakpointsForDimension1>
  Table_search_2D12 : Lookup_n-D  NumberOfTableDimensions=1  BreakpointsForDimension1=T2D_V_SFT_78_X  Table=T2D_V_SFT_78_Y  TableDataTypeStr=single  ExtrapMethod=Clip  UseLastTableValue=on  InternalRulePriority=Speed  OutDataTypeStr=single  RndMeth=Simplest  InputSameDT=on
      settings: AttributesFormatString=|
      | tbl = %<Table>
      | axis = %<BreakpointsForDimension1>
  Table_search_2D13 : Lookup_n-D  NumberOfTableDimensions=1  BreakpointsForDimension1=T2D_V_SFT_67_X  Table=T2D_V_SFT_67_Y  TableDataTypeStr=single  ExtrapMethod=Clip  UseLastTableValue=on  InternalRulePriority=Speed  OutDataTypeStr=single  RndMeth=Simplest  InputSameDT=on
      settings: AttributesFormatString=|
      | tbl = %<Table>
      | axis = %<BreakpointsForDimension1>
  Table_search_2D14 : Lookup_n-D  NumberOfTableDimensions=1  BreakpointsForDimension1=T2D_V_SFT_56_X  Table=T2D_V_SFT_56_Y  TableDataTypeStr=single  ExtrapMethod=Clip  UseLastTableValue=on  InternalRulePriority=Speed  OutDataTypeStr=single  RndMeth=Simplest  InputSameDT=on
      settings: AttributesFormatString=|
      | tbl = %<Table>
      | axis = %<BreakpointsForDimension1>
  Table_search_2D15 : Lookup_n-D  NumberOfTableDimensions=1  BreakpointsForDimension1=T2D_V_SFT_45_X  Table=T2D_V_SFT_45_Y  TableDataTypeStr=single  ExtrapMethod=Clip  UseLastTableValue=on  InternalRulePriority=Speed  OutDataTypeStr=single  RndMeth=Simplest  InputSameDT=on
      settings: AttributesFormatString=|
      | tbl = %<Table>
      | axis = %<BreakpointsForDimension1>
  Table_search_2D16 : Lookup_n-D  NumberOfTableDimensions=1  BreakpointsForDimension1=T2D_V_SFT_34_X  Table=T2D_V_SFT_34_Y  TableDataTypeStr=single  ExtrapMethod=Clip  UseLastTableValue=on  InternalRulePriority=Speed  OutDataTypeStr=single  RndMeth=Simplest  InputSameDT=on
      settings: AttributesFormatString=|
      | tbl = %<Table>
      | axis = %<BreakpointsForDimension1>
  Table_search_2D17 : Lookup_n-D  NumberOfTableDimensions=1  BreakpointsForDimension1=T2D_V_SFT_23_X  Table=T2D_V_SFT_23_Y  TableDataTypeStr=single  ExtrapMethod=Clip  UseLastTableValue=on  InternalRulePriority=Speed  OutDataTypeStr=single  RndMeth=Simplest  InputSameDT=on
      settings: AttributesFormatString=|
      | tbl = %<Table>
      | axis = %<BreakpointsForDimension1>
  Table_search_2D18 : Lookup_n-D  NumberOfTableDimensions=1  BreakpointsForDimension1=T2D_V_SFT_12_X  Table=T2D_V_SFT_12_Y  TableDataTypeStr=single  ExtrapMethod=Clip  UseLastTableValue=on  InternalRulePriority=Speed  OutDataTypeStr=single  RndMeth=Simplest  InputSameDT=on
      settings: AttributesFormatString=|
      | tbl = %<Table>
      | axis = %<BreakpointsForDimension1>
  Table_search_2D2 : Lookup_n-D  NumberOfTableDimensions=1  BreakpointsForDimension1=T2D_V_SFT_98_X  Table=T2D_V_SFT_98_Y  TableDataTypeStr=single  ExtrapMethod=Clip  UseLastTableValue=on  InternalRulePriority=Speed  OutDataTypeStr=single  RndMeth=Simplest  InputSameDT=on
      settings: AttributesFormatString=|
      | tbl = %<Table>
      | axis = %<BreakpointsForDimension1>
  Table_search_2D3 : Lookup_n-D  NumberOfTableDimensions=1  BreakpointsForDimension1=T2D_V_SFT_87_X  Table=T2D_V_SFT_87_Y  TableDataTypeStr=single  ExtrapMethod=Clip  UseLastTableValue=on  InternalRulePriority=Speed  OutDataTypeStr=single  RndMeth=Simplest  InputSameDT=on
      settings: AttributesFormatString=|
      | tbl = %<Table>
      | axis = %<BreakpointsForDimension1>
  Table_search_2D4 : Lookup_n-D  NumberOfTableDimensions=1  BreakpointsForDimension1=T2D_V_SFT_76_X  Table=T2D_V_SFT_76_Y  TableDataTypeStr=single  ExtrapMethod=Clip  UseLastTableValue=on  InternalRulePriority=Speed  OutDataTypeStr=single  RndMeth=Simplest  InputSameDT=on
      settings: AttributesFormatString=|
      | tbl = %<Table>
      | axis = %<BreakpointsForDimension1>
  Table_search_2D5 : Lookup_n-D  NumberOfTableDimensions=1  BreakpointsForDimension1=T2D_V_SFT_65_X  Table=T2D_V_SFT_65_Y  TableDataTypeStr=single  ExtrapMethod=Clip  UseLastTableValue=on  InternalRulePriority=Speed  OutDataTypeStr=single  RndMeth=Simplest  InputSameDT=on
      settings: AttributesFormatString=|
      | tbl = %<Table>
      | axis = %<BreakpointsForDimension1>
  Table_search_2D6 : Lookup_n-D  NumberOfTableDimensions=1  BreakpointsForDimension1=T2D_V_SFT_54_X  Table=T2D_V_SFT_54_Y  TableDataTypeStr=single  ExtrapMethod=Clip  UseLastTableValue=on  InternalRulePriority=Speed  OutDataTypeStr=single  RndMeth=Simplest  InputSameDT=on
      settings: AttributesFormatString=|
      | tbl = %<Table>
      | axis = %<BreakpointsForDimension1>
  Table_search_2D7 : Lookup_n-D  NumberOfTableDimensions=1  BreakpointsForDimension1=T2D_V_SFT_43_X  Table=T2D_V_SFT_43_Y  TableDataTypeStr=single  ExtrapMethod=Clip  UseLastTableValue=on  InternalRulePriority=Speed  OutDataTypeStr=single  RndMeth=Simplest  InputSameDT=on
      settings: AttributesFormatString=|
      | tbl = %<Table>
      | axis = %<BreakpointsForDimension1>
  Table_search_2D8 : Lookup_n-D  NumberOfTableDimensions=1  BreakpointsForDimension1=T2D_V_SFT_32_X  Table=T2D_V_SFT_32_Y  TableDataTypeStr=single  ExtrapMethod=Clip  UseLastTableValue=on  InternalRulePriority=Speed  OutDataTypeStr=single  RndMeth=Simplest  InputSameDT=on
      settings: AttributesFormatString=|
      | tbl = %<Table>
      | axis = %<BreakpointsForDimension1>
  Table_search_2D9 : Lookup_n-D  NumberOfTableDimensions=1  BreakpointsForDimension1=T2D_V_SFT_21_X  Table=T2D_V_SFT_21_Y  TableDataTypeStr=single  ExtrapMethod=Clip  UseLastTableValue=on  InternalRulePriority=Speed  OutDataTypeStr=single  RndMeth=Simplest  InputSameDT=on
      settings: AttributesFormatString=|
      | tbl = %<Table>
      | axis = %<BreakpointsForDimension1>
  gear_shift_map : Outport  OutDataTypeStr=int16
      settings: AttributesFormatString=シフトマップから算出されるギヤ段[-]
  wires:
  accel_position/1 -> Table_search_2D7/1, Table_search_2D8/1, Table_search_2D9/1, Table_search_2D10/1, Table_search_2D11/1, Table_search_2D12/1, Table_search_2D13/1, Table_search_2D14/1, Table_search_2D15/1, Table_search_2D16/1, Table_search_2D17/1, Table_search_2D18/1, Table_search_2D6/1, Table_search_2D5/1, Table_search_2D4/1, Table_search_2D3/1, Table_search_2D2/1, Table_search_2D1/1
  shifter_position/1 -> Relational Operator/1  "shifter_position"
  Relational Operator/1 -> Switch2/2
  Constant/1 -> Relational Operator/2
  Constant1/1 -> Switch2/1
  Switch2/1 -> gear_shift_map/1  "gear_shift_map"
  v_vehicle/1 -> Subsystem/2(v_vehicle), Subsystem1/2(v_vehicle), Subsystem2/2(v_vehicle), Subsystem3/2(v_vehicle1), Subsystem4/2(v_vehicle), Subsystem5/2(v_vehicle), Subsystem6/2(v_vehicle), Subsystem7/2(v_vehicle), Subsystem8/2(v_vehicle)  "v_vehicle"
  Table_search_2D1/1 -> Subsystem/4(v_shift_A9)  "ans"
  Table_search_2D10/1 -> Subsystem/3(v_shift_9A)  "ans"
  Subsystem/1(Out1) -> Switch2/3
  Subsystem1/1(Out1) -> Subsystem/5(elseif_Input5)
  Subsystem2/1(Out1) -> Subsystem1/5(elseif_Input5)
  Subsystem3/1(Out2) -> Subsystem2/5(elseif_Input5)
  Subsystem4/1(Out1) -> Subsystem3/5(elseif_Input1)
  Subsystem5/1(Out1) -> Subsystem4/5(elseif_Input5)
  Subsystem6/1(Out1) -> Subsystem5/5(elseif_Input5)
  Subsystem7/1(Out1) -> Subsystem6/5(elseif_Input5)
  Subsystem8/1(Out1) -> Subsystem7/5(elseif_Input5)
  Table_search_2D2/1 -> Subsystem1/4(v_shift_98)  "ans"
  Table_search_2D3/1 -> Subsystem2/4(v_shift_87)  "ans"
  Table_search_2D4/1 -> Subsystem3/4(v_shift_2)  "ans"
  Table_search_2D5/1 -> Subsystem4/4(v_shift_65)  "ans"
  Table_search_2D6/1 -> Subsystem5/4(v_shift_54)  "ans"
  Table_search_2D7/1 -> Subsystem6/4(v_shift_43)  "ans"
  Table_search_2D8/1 -> Subsystem7/4(v_shift_32)  "ans"
  Table_search_2D11/1 -> Subsystem1/3(v_shift_89)  "ans"
  Table_search_2D12/1 -> Subsystem2/3(v_shift_78)  "ans"
  Table_search_2D13/1 -> Subsystem3/3(v_shift_1)  "ans"
  Table_search_2D14/1 -> Subsystem4/3(v_shift_56)  "ans"
  Table_search_2D15/1 -> Subsystem5/3(v_shift_45)  "ans"
  Table_search_2D16/1 -> Subsystem6/3(v_shift_34)  "ans"
  Table_search_2D17/1 -> Subsystem7/3(v_shift_23)  "ans"
  Table_search_2D18/1 -> Subsystem8/3(v_shift_12)  "ans"
  Constant2/1 -> Subsystem8/5(elseif_Input5)
  Table_search_2D9/1 -> Subsystem8/4(v_shift_21)  "ans"
  gear_shift_map_old/1 -> Subsystem/1(gear_shift_map_old), Subsystem1/1(gear_shift_map_old), Subsystem2/1(gear_shift_map_old), Subsystem3/1(gear_shift_map_old1), Subsystem4/1(gear_shift_map_old), Subsystem5/1(gear_shift_map_old), Subsystem6/1(gear_shift_map_old), Subsystem7/1(gear_shift_map_old), Subsystem8/1(gear_shift_map_old)  "gear_shift_map_old"
